simulink model "mdl_SMO_spm_foc_plus_inv"  (R2022b)
settings: Solver=ode3  StartTime=0.0  StopTime=0.4  FixedStep=1e-6  RelTol=1e-3  EnableMultiTasking=on
undefined symbols (not defined in the file): Ls, Rs
libraries: slpidlib x3, spsDCVoltageSourceLib x1, spsGroundLib x1, spsTriangleGeneratorLib x1, spsPermanentMagnetSynchronousMachineLib x1, spsThreePhaseVIMeasurementLib x1, spsUniversalBridgeLib x1, spspowerguiLib x1
settings Model: Creator=jack  LastModifiedBy=jackyeh
settings DebuggingCC: SolverPrmCheckMsg=warning  StateNameClashWarn=warning

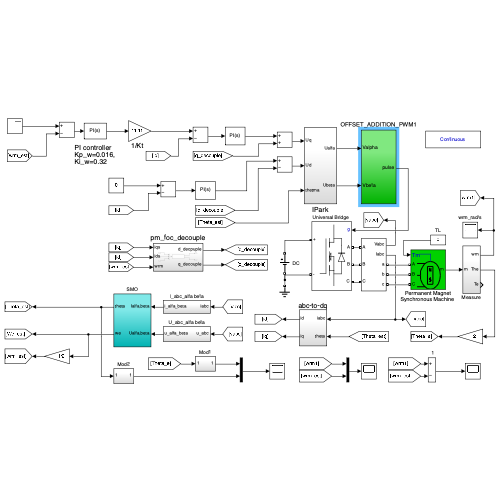
[thumbnail: Simulink's stored preview of the top-level diagram]
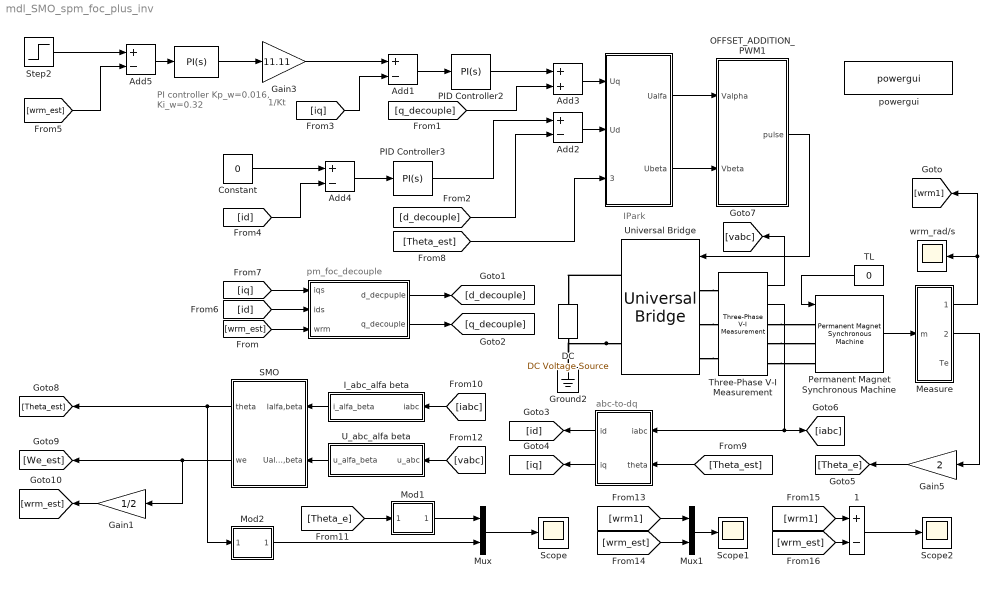
== system mdl_SMO_spm_foc_plus_inv ==
  note: abc-to-dq
  note: IPark
  note: pm_foc_decouple
  note: PI controller
      | Kp_w=0.016, Ki_w=0.32
  note: 1/Kt
  "   " : slpidlib/PID Controller  Controller=PI  Form=Parallel  TimeDomain=Continuous-time  UseExternalTs=off  SampleTime=-1  IntegratorMethod=Forward Euler  FilterMethod=Forward Euler  ControllerParametersSource=internal  P=0.016  I=0.32  UseKiTs=off  D=0  N=100  UseFilter=on  TunerSelectOption=Transfer Function Based (PID Tuner App)  InitialConditionSource=internal  InitialConditionForIntegrator=0  InitialConditionForFilter=0  DifferentiatorICPrevScaledInput=0  ExternalReset=none  TrackingMode=off  Kt=1  LimitOutput=off  SatLimitsSource=internal  UpperSaturationLimit=inf  LowerSaturationLimit=-inf  LinearizeAsGain=on  AntiWindupMode=none  Kb=1  LimitIntegrator=off  UpperIntegratorSaturationLimit=inf  LowerIntegratorSaturationLimit=-inf  POutMin=[]  POutMax=[]  IOutMin=[]  IOutMax=[]  DOutMin=[]  DOutMax=[]  NOutMin=[]  NOutMax=[]  SumOutMin=[]  SumOutMax=[]  SaturationOutMin=[]  SaturationOutMax=[]  PParamMin=[]  PParamMax=[]  IParamMin=[]  IParamMax=[]  DParamMin=[]  DParamMax=[]  NParamMin=[]  NParamMax=[]  KbParamMin=[]  KbParamMax=[]  KtParamMin=[]  KtParamMax=[]  KbOutMin=[]  KbOutMax=[]  KtOutMin=[]  KtOutMax=[]  IntegratorOutMin=[]  IntegratorOutMax=[]  FilterOutMin=[]  FilterOutMax=[]  SumI1OutMin=[]  SumI1OutMax=[]  SumI2OutMin=[]  SumI2OutMax=[]  SumI3OutMin=[]  SumI3OutMax=[]  SumI4OutMin=[]  SumI4OutMax=[]  SumDOutMin=[]  SumDOutMax=[]  DifferentiatorOutMin=[]  DifferentiatorOutMax=[]  FilterDiffOutCoefMin=[]  FilterDiffOutCoefMax=[]  ReciprocalOutMin=[]  ReciprocalOutMax=[]  SumDenOutMin=[]  SumDenOutMax=[]  SumNumOutMin=[]  SumNumOutMax=[]  DivideOutMin=[]  DivideOutMax=[]  UdiffTsProdOutMin=[]  UdiffTsProdOutMax=[]  NTsProdOutMin=[]  NTsProdOutMax=[]  UintegralTsProdOutMin=[]  UintegralTsProdOutMax=[]  UngainTsProdOutMin=[]  UngainTsProdOutMax=[]  ClampingZeroOutDataTypeStr=Inherit: Inherit via back propagation  ClampingZeroOutMin=[]  ClampingZeroOutMax=[]  FilterDenConstantOutDataTypeStr=Inherit: Inherit via back propagation  FilterDenConstantOutMin=[]  FilterDenConstantOutMax=[]  PCopyOutDataTypeStr=Inherit: Inherit via back propagation  PCopyOutMin=[]  PCopyOutMax=[]  NCopyOutDataTypeStr=Inherit: Inherit via back propagation  NCopyOutMin=[]  NCopyOutMax=[]  IntegratorContinuousStateAttributes=''  IntegratorStateMustResolveToSignalObject=off  IntegratorRTWStateStorageClass=Auto  FilterContinuousStateAttributes=''  FilterStateMustResolveToSignalObject=off  FilterRTWStateStorageClass=Auto  ParallelPVariant=InternalParameters  IdealPVariant=Disabled  IVariant=InternalParameters  DVariant=Disabled  IntegratorVariant=Continuous  SatVariant=Disabled  AWVariant=Passthrough  PCopyVariant=Disabled  TRVariant=Disabled  FdbkBlocksVariant=Forward  IdealPFdbkVariant=Disabled  SatFdbkVariant=Disabled  DerivativeFilterVariant=Disabled  NVariant=Disabled  NCopyVariant=Disabled_SignalSpec  FilterICVariant=Disabled  IntegratorICVariant=InternalICs  ExternalResetVariant=Disabled  TRSumVariant=Passthrough  SumFdbkVariant=Disabled  SumVariant=Sum_PI  TsampFilterVariant=InternalTs  TsampNgainVariant=Passthrough  TsampIntegralVariant=Passthrough  ExternalSaturationOutDataTypeStr=Inherit: Same as second input
  "    " : Subsystem
  "     " : Subsystem
  "      " : Subsystem
  "  1" : Sum  Inputs=+-
  Add{1..2,4..5} (4 alike) : Sum  Inputs=+-
  Add3 : Sum
  Constant : Constant  Value=0
  "DC " : spsDCVoltageSourceLib/DC Voltage Source  Amplitude=311  Measurements=None
  Gain1 : Gain  Gain=1/2
  Gain3 : Gain  Gain=11.11
  Gain5 : Gain  Gain=2
  Ground2 : spsGroundLib/Ground  LConnTagsString=a
  I_abc_alfa beta : Subsystem
  Measure : Subsystem
  Mod1 : Subsystem
  Mod2 : Subsystem
  Mux : Mux  Inputs=2
  Mux1 : Mux  Inputs=2
  OFFSET_ADDITION_PWM1 : Subsystem
  PID Controller2 : slpidlib/PID Controller  Controller=PI  Form=Parallel  TimeDomain=Continuous-time  UseExternalTs=off  SampleTime=-1  IntegratorMethod=Forward Euler  FilterMethod=Forward Euler  ControllerParametersSource=internal  P=5.7  I=1200  UseKiTs=off  D=0  N=100  UseFilter=on  TunerSelectOption=Transfer Function Based (PID Tuner App)  InitialConditionSource=internal  InitialConditionForIntegrator=0  InitialConditionForFilter=0  DifferentiatorICPrevScaledInput=0  ExternalReset=none  TrackingMode=off  Kt=1  LimitOutput=off  SatLimitsSource=internal  UpperSaturationLimit=inf  LowerSaturationLimit=-inf  LinearizeAsGain=on  AntiWindupMode=none  Kb=1  LimitIntegrator=off  UpperIntegratorSaturationLimit=inf  LowerIntegratorSaturationLimit=-inf  POutMin=[]  POutMax=[]  IOutMin=[]  IOutMax=[]  DOutMin=[]  DOutMax=[]  NOutMin=[]  NOutMax=[]  SumOutMin=[]  SumOutMax=[]  SaturationOutMin=[]  SaturationOutMax=[]  PParamMin=[]  PParamMax=[]  IParamMin=[]  IParamMax=[]  DParamMin=[]  DParamMax=[]  NParamMin=[]  NParamMax=[]  KbParamMin=[]  KbParamMax=[]  KtParamMin=[]  KtParamMax=[]  KbOutMin=[]  KbOutMax=[]  KtOutMin=[]  KtOutMax=[]  IntegratorOutMin=[]  IntegratorOutMax=[]  FilterOutMin=[]  FilterOutMax=[]  SumI1OutMin=[]  SumI1OutMax=[]  SumI2OutMin=[]  SumI2OutMax=[]  SumI3OutMin=[]  SumI3OutMax=[]  SumI4OutMin=[]  SumI4OutMax=[]  SumDOutMin=[]  SumDOutMax=[]  DifferentiatorOutMin=[]  DifferentiatorOutMax=[]  FilterDiffOutCoefMin=[]  FilterDiffOutCoefMax=[]  ReciprocalOutMin=[]  ReciprocalOutMax=[]  SumDenOutMin=[]  SumDenOutMax=[]  SumNumOutMin=[]  SumNumOutMax=[]  DivideOutMin=[]  DivideOutMax=[]  UdiffTsProdOutMin=[]  UdiffTsProdOutMax=[]  NTsProdOutMin=[]  NTsProdOutMax=[]  UintegralTsProdOutMin=[]  UintegralTsProdOutMax=[]  UngainTsProdOutMin=[]  UngainTsProdOutMax=[]  ClampingZeroOutDataTypeStr=Inherit: Inherit via back propagation  ClampingZeroOutMin=[]  ClampingZeroOutMax=[]  FilterDenConstantOutDataTypeStr=Inherit: Inherit via back propagation  FilterDenConstantOutMin=[]  FilterDenConstantOutMax=[]  PCopyOutDataTypeStr=Inherit: Inherit via back propagation  PCopyOutMin=[]  PCopyOutMax=[]  NCopyOutDataTypeStr=Inherit: Inherit via back propagation  NCopyOutMin=[]  NCopyOutMax=[]  IntegratorContinuousStateAttributes=''  IntegratorStateMustResolveToSignalObject=off  IntegratorRTWStateStorageClass=Auto  FilterContinuousStateAttributes=''  FilterStateMustResolveToSignalObject=off  FilterRTWStateStorageClass=Auto  ParallelPVariant=InternalParameters  IdealPVariant=Disabled  IVariant=InternalParameters  DVariant=Disabled  IntegratorVariant=Continuous  SatVariant=Disabled  AWVariant=Passthrough  PCopyVariant=Disabled  TRVariant=Disabled  FdbkBlocksVariant=Forward  IdealPFdbkVariant=Disabled  SatFdbkVariant=Disabled  DerivativeFilterVariant=Disabled  NVariant=Disabled  NCopyVariant=Disabled_SignalSpec  FilterICVariant=Disabled  IntegratorICVariant=InternalICs  ExternalResetVariant=Disabled  TRSumVariant=Passthrough  SumFdbkVariant=Disabled  SumVariant=Sum_PI  TsampFilterVariant=InternalTs  TsampNgainVariant=Passthrough  TsampIntegralVariant=Passthrough  ExternalSaturationOutDataTypeStr=Inherit: Same as second input
  PID Controller3 : slpidlib/PID Controller  Controller=PI  Form=Parallel  TimeDomain=Continuous-time  UseExternalTs=off  SampleTime=-1  IntegratorMethod=Forward Euler  FilterMethod=Forward Euler  ControllerParametersSource=internal  P=5.7  I=1200  UseKiTs=off  D=0  N=100  UseFilter=on  TunerSelectOption=Transfer Function Based (PID Tuner App)  InitialConditionSource=internal  InitialConditionForIntegrator=0  InitialConditionForFilter=0  DifferentiatorICPrevScaledInput=0  ExternalReset=none  TrackingMode=off  Kt=1  LimitOutput=off  SatLimitsSource=internal  UpperSaturationLimit=inf  LowerSaturationLimit=-inf  LinearizeAsGain=on  AntiWindupMode=none  Kb=1  LimitIntegrator=off  UpperIntegratorSaturationLimit=inf  LowerIntegratorSaturationLimit=-inf  POutMin=[]  POutMax=[]  IOutMin=[]  IOutMax=[]  DOutMin=[]  DOutMax=[]  NOutMin=[]  NOutMax=[]  SumOutMin=[]  SumOutMax=[]  SaturationOutMin=[]  SaturationOutMax=[]  PParamMin=[]  PParamMax=[]  IParamMin=[]  IParamMax=[]  DParamMin=[]  DParamMax=[]  NParamMin=[]  NParamMax=[]  KbParamMin=[]  KbParamMax=[]  KtParamMin=[]  KtParamMax=[]  KbOutMin=[]  KbOutMax=[]  KtOutMin=[]  KtOutMax=[]  IntegratorOutMin=[]  IntegratorOutMax=[]  FilterOutMin=[]  FilterOutMax=[]  SumI1OutMin=[]  SumI1OutMax=[]  SumI2OutMin=[]  SumI2OutMax=[]  SumI3OutMin=[]  SumI3OutMax=[]  SumI4OutMin=[]  SumI4OutMax=[]  SumDOutMin=[]  SumDOutMax=[]  DifferentiatorOutMin=[]  DifferentiatorOutMax=[]  FilterDiffOutCoefMin=[]  FilterDiffOutCoefMax=[]  ReciprocalOutMin=[]  ReciprocalOutMax=[]  SumDenOutMin=[]  SumDenOutMax=[]  SumNumOutMin=[]  SumNumOutMax=[]  DivideOutMin=[]  DivideOutMax=[]  UdiffTsProdOutMin=[]  UdiffTsProdOutMax=[]  NTsProdOutMin=[]  NTsProdOutMax=[]  UintegralTsProdOutMin=[]  UintegralTsProdOutMax=[]  UngainTsProdOutMin=[]  UngainTsProdOutMax=[]  ClampingZeroOutDataTypeStr=Inherit: Inherit via back propagation  ClampingZeroOutMin=[]  ClampingZeroOutMax=[]  FilterDenConstantOutDataTypeStr=Inherit: Inherit via back propagation  FilterDenConstantOutMin=[]  FilterDenConstantOutMax=[]  PCopyOutDataTypeStr=Inherit: Inherit via back propagation  PCopyOutMin=[]  PCopyOutMax=[]  NCopyOutDataTypeStr=Inherit: Inherit via back propagation  NCopyOutMin=[]  NCopyOutMax=[]  IntegratorContinuousStateAttributes=''  IntegratorStateMustResolveToSignalObject=off  IntegratorRTWStateStorageClass=Auto  FilterContinuousStateAttributes=''  FilterStateMustResolveToSignalObject=off  FilterRTWStateStorageClass=Auto  ParallelPVariant=InternalParameters  IdealPVariant=Disabled  IVariant=InternalParameters  DVariant=Disabled  IntegratorVariant=Continuous  SatVariant=Disabled  AWVariant=Passthrough  PCopyVariant=Disabled  TRVariant=Disabled  FdbkBlocksVariant=Forward  IdealPFdbkVariant=Disabled  SatFdbkVariant=Disabled  DerivativeFilterVariant=Disabled  NVariant=Disabled  NCopyVariant=Disabled_SignalSpec  FilterICVariant=Disabled  IntegratorICVariant=InternalICs  ExternalResetVariant=Disabled  TRSumVariant=Passthrough  SumFdbkVariant=Disabled  SumVariant=Sum_PI  TsampFilterVariant=InternalTs  TsampNgainVariant=Passthrough  TsampIntegralVariant=Passthrough  ExternalSaturationOutDataTypeStr=Inherit: Same as second input
  "Permanent Magnet Synchronous Machine " : spsPermanentMagnetSynchronousMachineLib/Permanent Magnet Synchronous Machine  NbPhases=3  FluxDistribution=Sinusoidal  RotorType=Salient-pole  MechanicalLoad=Torque Tm  PresetModel=No  ShowDetailedParameters=on  MeasurementBus=off  Resistance=1.2  Inductance=8.5e-3  dqInductances=[5.7e-3, 5.7e-3]  La=5.7e-3  MachineConstant=Flux linkage established by magnets (V.s)  Flux=0.03  VoltageCst=10.8828  TorqueCst=0.09  Flat=120  Mechanical="[0.00016  0 2]"  PolePairs=4  InitialConditions=[0,0, 0,0]  InitialConditions5ph=[0 0 0 0 0 0]  RefAngle=Aligned with phase A axis (original Park)  IterativeDiscreteModel=Trapezoidal non iterative  TsBlock=-1  TsPowergui=0
  SMO : Subsystem
  Scope : Scope
  Scope1 : Scope
  Scope2 : Scope
  Step2 : Step  Time=0  After=100  SampleTime=0
  TL : Constant  Value=0
  Three-Phase V-I Measurement : spsThreePhaseVIMeasurementLib/Three-Phase V-I Measurement  VoltageMeasurement=phase-to-ground  SetLabelV=off  LabelV=Vabc  Vpu=off  VpuLL=off  CurrentMeasurement=yes  SetLabelI=off  LabelI=Iabc  Ipu=off  Pbase=100e6  Vbase=500e3  OutputType=Complex  PhasorSimulation=off  PSBequivalent=0
  U_abc_alfa beta : Subsystem
  "Universal Bridge " : spsUniversalBridgeLib/Universal Bridge  Arms=3  SnubberResistance=1e5  SnubberCapacitance=inf  Device=MOSFET / Diodes  Ron=1e-3  Lon=0  ForwardVoltages="[  0  0  ]"  ForwardVoltage=0  GTOparameters=[ 10e-6 , 20e-6 ]  IGBTparameters=[ 1e-6 , 2e-6 ]  Measurements=None  Measurements_2=None  converterType=Rectifier
  powergui : spspowerguiLib/powergui  Priority=1  SimulationMode=Continuous  SampleTime=50e-6  frequency=60  Iterations=50  frequencyindice=0  Pbase=100e6  ErrMax=1e-4  UnitsV=kV  UnitsW=MW  buscounter=0  FunctionMessages=off  echomessages=off  EnableUseOfTLC=off  CurrentSourceSwitches=off  DisableSnubberDevices=off  DisableRonSwitches=off  DisableVfSwitches=off  DisplayEquations=off  AutomaticDiscreteSolvers=off  SolverType=Tustin/Backward Euler (TBE)  Interpol=off  ExternalGateDelay=off  methode=off  Ts=100  x0status=blocks  SPID=off  SwTol=0  HookPort=off  NonlinearTolerance=1e-4  nMaxIteration=100  ContinueOnMaxIteration=off  RestoreLinks=warning  ResistiveCurrentMeasurement=off  Frange=[0:2:500]  Ylog=off  Xlog=on  ShowGrid=off  save=off  variable=ZData  structure=0  ZoomFFT=off  StartTime=0.0  cycles=1  DisplayStyle=1  fundamental=60  FreqAxis=off  MaxFrequency=1000  frequencyindicesteady=1  RmsSteady=1  display=off
  wrm_rad/s : Scope
  wires:
  "   "/1 -> Gain3/1
  Add1/1 -> PID Controller2/1
  Constant/1 -> Add4/1
  Add4/1 -> PID Controller3/1
  Add5/1 -> "   "/1
  "Permanent Magnet Synchronous Machine "/1 -> Measure/1(m)
  OFFSET_ADDITION_PWM1/1(pulse) -> "Universal Bridge "/1
  "     "/1(Ualfa) -> OFFSET_ADDITION_PWM1/1(Valpha)
  "     "/2(Ubeta) -> OFFSET_ADDITION_PWM1/2(Vbeta)
  Three-Phase V-I Measurement/2 -> [iabc], "      "/1(iabc)
  Measure/2(The) -> Gain5/1
  Measure/1(wm) -> [wrm1], wrm_rad/s/1
  PID Controller3/1 -> Add2/1
  PID Controller2/1 -> Add3/1
  Add3/1 -> "     "/1(Uq)
  Add2/1 -> "     "/2(Ud)
  [wrm_est] -> "    "/3(wrm)
  Gain3/1 -> Add1/1
  Step2/1 -> Add5/1
  TL/1 -> "Permanent Magnet Synchronous Machine "/1
  "    "/1(d_decpuple) -> [d_decouple]
  "    "/2(q_decouple) -> [q_decouple]
  "      "/1(id) -> [id]
  "      "/2(iq) -> [iq]
  [iq] -> Add1/2
  [id] -> Add4/2
  [wrm_est] -> Add5/2
  [iq] -> "    "/1(iqs)
  [id] -> "    "/2(ids)
  [Theta_est] -> "     "/3(thetma)
  [Theta_est] -> "      "/2(theta)
  I_abc_alfa beta/1(i_alfa_beta) -> SMO/1(Ialfa,beta)
  U_abc_alfa beta/1(u_alfa_beta) -> SMO/2(Ualfa,beta)
  Three-Phase V-I Measurement/1 -> [vabc]
  [iabc] -> I_abc_alfa beta/1(iabc)
  [vabc] -> U_abc_alfa beta/1(u_abc)
  SMO/2(we) -> Gain1/1, [We_est]
  Gain1/1 -> [wrm_est]
  Mux/1 -> Scope/1
  Gain5/1 -> [Theta_e]
  [q_decouple] -> Add3/2
  [d_decouple] -> Add2/2
  SMO/1(theta) -> [Theta_est], Mod2/1(In1)
  [Theta_e] -> Mod1/1(In1)
  Mod1/1(Out1) -> Mux/1
  [wrm1] -> Mux1/1
  [wrm_est] -> Mux1/2
  Mux1/1 -> Scope1/1
  [wrm1] -> "  1"/1
  [wrm_est] -> "  1"/2
  "  1"/1 -> Scope2/1
  Mod2/1(Out1) -> Mux/2
  connections:
  "Universal Bridge "/RConn2 -- Ground2/LConn1 -- "DC "/LConn1
  "Universal Bridge "/LConn1 -- Three-Phase V-I Measurement/LConn1
  "Universal Bridge "/LConn3 -- Three-Phase V-I Measurement/LConn3
  Three-Phase V-I Measurement/RConn3 -- "Permanent Magnet Synchronous Machine "/LConn3
  Three-Phase V-I Measurement/RConn1 -- "Permanent Magnet Synchronous Machine "/LConn1
  Three-Phase V-I Measurement/RConn2 -- "Permanent Magnet Synchronous Machine "/LConn2
  "Universal Bridge "/RConn1 -- "DC "/RConn1
  "Universal Bridge "/LConn2 -- Three-Phase V-I Measurement/LConn2

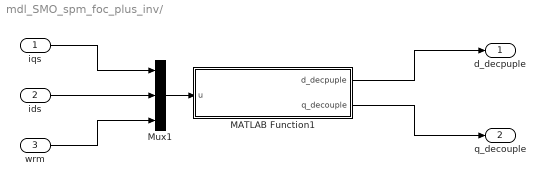
== system mdl_SMO_spm_foc_plus_inv/     ==
  iqs : Inport
  ids : Inport  Port=2
  wrm : Inport  Port=3
  MATLAB Function1 : MATLAB Function  TreatAsAtomicUnit=on
  Mux1 : Mux  Inputs=3
  d_decpuple : Outport
  q_decouple : Outport  Port=2
  wires:
  iqs/1 -> Mux1/1
  MATLAB Function1/1(d_decpuple) -> d_decpuple/1
  ids/1 -> Mux1/2
  Mux1/1 -> MATLAB Function1/1(u)
  MATLAB Function1/2(q_decouple) -> q_decouple/1
  wrm/1 -> Mux1/3

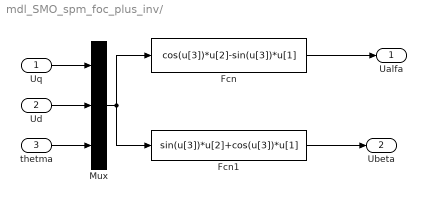
== system mdl_SMO_spm_foc_plus_inv/      ==
  Uq : Inport
  Ud : Inport  Port=2
  thetma : Inport  Port=3
  Fcn : Fcn  Expr=cos(u[3])*u[2]-sin(u[3])*u[1]
  Fcn1 : Fcn  Expr=sin(u[3])*u[2]+cos(u[3])*u[1]
  Mux : Mux  Inputs=3
  Ualfa : Outport
  Ubeta : Outport  Port=2
  wires:
  Uq/1 -> Mux/1
  Ud/1 -> Mux/2
  thetma/1 -> Mux/3
  Mux/1 -> Fcn/1, Fcn1/1
  Fcn/1 -> Ualfa/1
  Fcn1/1 -> Ubeta/1

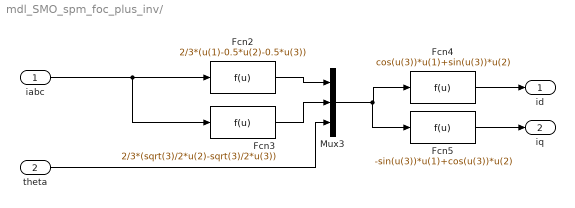
== system mdl_SMO_spm_foc_plus_inv/       ==
  iabc : Inport
  theta : Inport  Port=2
  Fcn2 : Fcn  Expr=2/3*(u(1)-0.5*u(2)-0.5*u(3))
  Fcn3 : Fcn  Expr=2/3*(sqrt(3)/2*u(2)-sqrt(3)/2*u(3))
  Fcn4 : Fcn  Expr=cos(u(3))*u(1)+sin(u(3))*u(2)
  Fcn5 : Fcn  Expr=-sin(u(3))*u(1)+cos(u(3))*u(2)
  Mux3 : Mux  Inputs=3
  id : Outport
  iq : Outport  Port=2
  wires:
  iabc/1 -> Fcn3/1, Fcn2/1
  Fcn2/1 -> Mux3/1
  Fcn3/1 -> Mux3/2
  theta/1 -> Mux3/3
  Mux3/1 -> Fcn5/1, Fcn4/1
  Fcn4/1 -> id/1
  Fcn5/1 -> iq/1

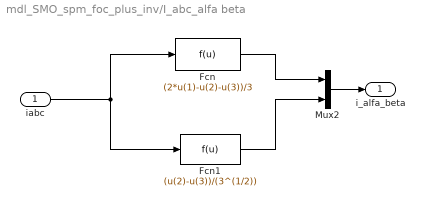
== system mdl_SMO_spm_foc_plus_inv/I_abc_alfa beta ==
  iabc : Inport
  Fcn : Fcn  Expr=(2*u(1)-u(2)-u(3))/3
  Fcn1 : Fcn  Expr=(u(2)-u(3))/(3^(1/2))
  Mux2 : Mux  Inputs=2
  i_alfa_beta : Outport
  wires:
  iabc/1 -> Fcn/1, Fcn1/1
  Mux2/1 -> i_alfa_beta/1
  Fcn/1 -> Mux2/1
  Fcn1/1 -> Mux2/2

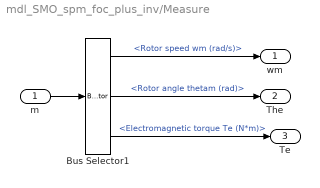
== system mdl_SMO_spm_foc_plus_inv/Measure ==
  m : Inport
  Bus Selector1 : BusSelector  OutputSignals=Rotor speed wm (rad/s),Rotor angle thetam (rad),Electromagnetic torque Te (N*m)
  wm : Outport
  The : Outport  Port=2
  Te : Outport  Port=3
  wires:
  Bus Selector1/2 -> The/1  "<Rotor angle thetam (rad)>"
  Bus Selector1/3 -> Te/1  "<Electromagnetic torque Te (N*m)>"
  m/1 -> Bus Selector1/1
  Bus Selector1/1 -> wm/1  "<Rotor speed wm (rad/s)>"

== system mdl_SMO_spm_foc_plus_inv/Mod1 ==
  In1 : Inport
  Constant1 : Constant  Value=pi
  Math Function : Math  Operator=mod  SignedPower=on
  Out1 : Outport
  wires:
  In1/1 -> Math Function/1
  Math Function/1 -> Out1/1
  Constant1/1 -> Math Function/2

== system mdl_SMO_spm_foc_plus_inv/Mod2 ==
  In1 : Inport
  Constant1 : Constant  Value=pi
  Math Function : Math  Operator=mod  SignedPower=on
  Out1 : Outport
  wires:
  Constant1/1 -> Math Function/2
  Math Function/1 -> Out1/1
  In1/1 -> Math Function/1

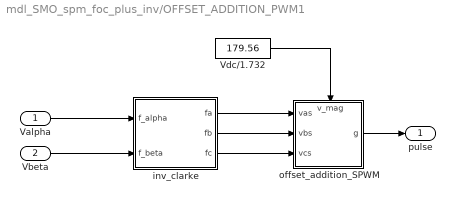
== system mdl_SMO_spm_foc_plus_inv/OFFSET_ADDITION_PWM1 ==
  Valpha : Inport
  Vbeta : Inport  Port=2
  Vdc/1.732 : Constant  Value=179.56
  inv_clarke : Subsystem
  offset_addition_SPWM : Subsystem
      settings: PortSchema="{\"entries\":[{\"content\":{\"sides\":[{\"content\":{\"connectorIds\":[\"In1\",\"In2\",\"In3\"]},\"type\":\"ConnectorPlacement.EquallySpacedRectSide\",\"uuid\":\"bd7bea3a-7add-49ec-8b52-f68dbb33beea\"},{\"content\":{\"connectorIds\":[\"Out1\"],\"side\":\"RIGHT\"},\"type\":\"ConnectorPlacement.EquallySpacedRectSide\",\"uuid\":\"aa5e81bc-27af-49d7-8d73-7e78ac021e04\"},{\"content\":{\"connectorIds\":[\"In4\"],\"side\":\"TOP\"},\"type\":\"ConnectorPlacement.EquallySpacedRectSide\",\"uuid\":\"5bcd18e6-6f27-4bab-991b-2041f8ef0a25\"}]},\"type\":\"ConnectorPlacement.EquallySpacedConnector\",\"uuid\":\"27ed4ada-ba8b-4440-bbdb-1c3a657b0505\"}],\"packageUris\":[\"http://schema.mathworks.com/mf0/Connector/R2020b\"],\"version\":\"1.0\"}"
  pulse : Outport
  wires:
  Valpha/1 -> inv_clarke/1(f_alpha)
  Vbeta/1 -> inv_clarke/2(f_beta)
  inv_clarke/1(fa) -> offset_addition_SPWM/1(vas)
  inv_clarke/2(fb) -> offset_addition_SPWM/2(vbs)
  inv_clarke/3(fc) -> offset_addition_SPWM/3(vcs)
  offset_addition_SPWM/1(g) -> pulse/1
  Vdc/1.732/1 -> offset_addition_SPWM/4(v_mag)

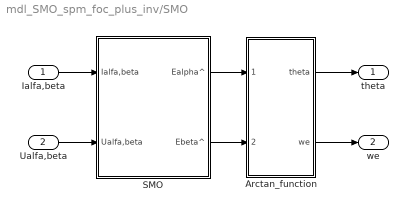
== system mdl_SMO_spm_foc_plus_inv/SMO ==
  Ialfa,beta : Inport
  Ualfa,beta : Inport  Port=2
  Arctan_function : Subsystem
  SMO : Subsystem
  theta : Outport
  we : Outport  Port=2
  wires:
  Ualfa,beta/1 -> SMO/2(Ualfa,beta)
  Ialfa,beta/1 -> SMO/1(Ialfa,beta)
  SMO/1(Ealpha^) -> Arctan_function/1(Ealpha^)
  SMO/2(Ebeta^) -> Arctan_function/2(Ebeta^)
  Arctan_function/1(theta) -> theta/1
  Arctan_function/2(we) -> we/1

== system mdl_SMO_spm_foc_plus_inv/U_abc_alfa beta ==
  u_abc : Inport
  Fcn : Fcn  Expr=(2*u(1)-u(2)-u(3))/3
  Fcn1 : Fcn  Expr=(u(2)-u(3))/(3^(1/2))
  Mux2 : Mux  Inputs=2
  u_alfa_beta : Outport
  wires:
  u_abc/1 -> Fcn/1, Fcn1/1
  Mux2/1 -> u_alfa_beta/1
  Fcn/1 -> Mux2/1
  Fcn1/1 -> Mux2/2

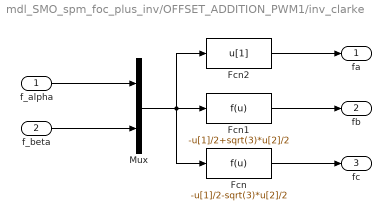
== system mdl_SMO_spm_foc_plus_inv/OFFSET_ADDITION_PWM1/inv_clarke ==
  f_alpha : Inport
  f_beta : Inport  Port=2
  Fcn : Fcn  Expr=-u[1]/2-sqrt(3)*u[2]/2
  Fcn1 : Fcn  Expr=-u[1]/2+sqrt(3)*u[2]/2
  Fcn2 : Fcn  Expr=u[1]
  Mux : Mux  Inputs=2
  fa : Outport
  fb : Outport  Port=2
  fc : Outport  Port=3
  wires:
  Mux/1 -> Fcn2/1, Fcn1/1, Fcn/1
  f_alpha/1 -> Mux/1
  f_beta/1 -> Mux/2
  Fcn2/1 -> fa/1
  Fcn1/1 -> fb/1
  Fcn/1 -> fc/1

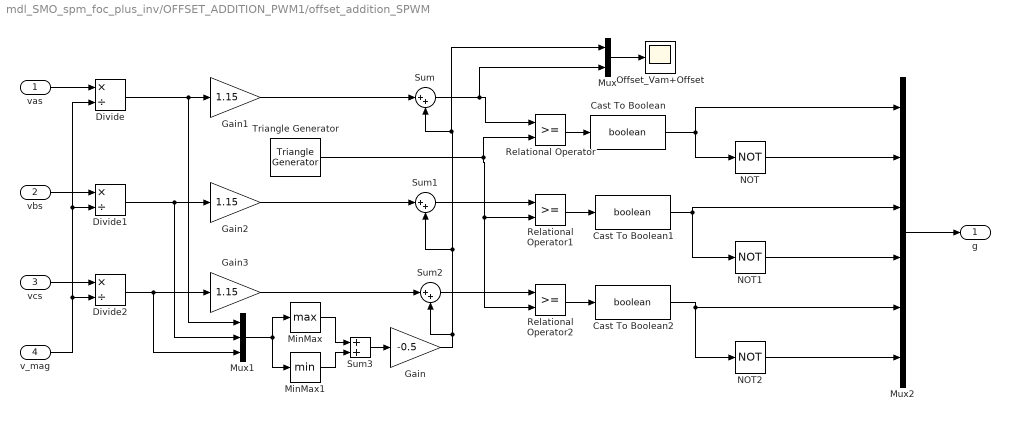
== system mdl_SMO_spm_foc_plus_inv/OFFSET_ADDITION_PWM1/offset_addition_SPWM ==
  vas : Inport
  vbs : Inport  Port=2
  vcs : Inport  Port=3
  v_mag : Inport  Port=4
  Cast To Boolean : DataTypeConversion  OutDataTypeStr=boolean  SaturateOnIntegerOverflow=off  RndMeth=Floor
  Cast To Boolean1 : DataTypeConversion  OutDataTypeStr=boolean  SaturateOnIntegerOverflow=off  RndMeth=Floor
  Cast To Boolean2 : DataTypeConversion  OutDataTypeStr=boolean  SaturateOnIntegerOverflow=off  RndMeth=Floor
  Divide : Product  Inputs=*/
  Divide1 : Product  Inputs=*/
  Divide2 : Product  Inputs=*/
  Gain : Gain  Gain=-0.5
  Gain1 : Gain  Gain=1.15
  Gain2 : Gain  Gain=1.15
  Gain3 : Gain  Gain=1.15
  MinMax : MinMax  Function=max
  MinMax1 : MinMax
  Mux : Mux  Inputs=2
  Mux1 : Mux  Inputs=3
  Mux2 : Mux  Inputs=6
  NOT : Logic  Operator=NOT  IconShape=distinctive  AllPortsSameDT=off  OutDataTypeStr=boolean
  NOT1 : Logic  Operator=NOT  IconShape=distinctive  AllPortsSameDT=off  OutDataTypeStr=boolean
  NOT2 : Logic  Operator=NOT  IconShape=distinctive  AllPortsSameDT=off  OutDataTypeStr=boolean
  Offset_Vam+Offset : Scope
  Relational Operator : RelationalOperator  OutDataTypeStr=boolean  RndMeth=Simplest  InputSameDT=off
  Relational Operator1 : RelationalOperator  OutDataTypeStr=boolean  RndMeth=Simplest  InputSameDT=off
  Relational Operator2 : RelationalOperator  OutDataTypeStr=boolean  RndMeth=Simplest  InputSameDT=off
  Sum : Sum  Inputs=|++
  Sum1 : Sum  Inputs=|++
  Sum2 : Sum  Inputs=|++
  Sum3 : Sum
  Triangle Generator : spsTriangleGeneratorLib/Triangle Generator  Freq=10000  Phase=90  Ts=0
  g : Outport
  wires:
  NOT/1 -> Mux2/2
  Relational Operator/1 -> Cast To Boolean/1
  Cast To Boolean/1 -> Mux2/1, NOT/1
  Triangle Generator/1 -> Relational Operator2/2, Relational Operator1/2, Relational Operator/2
  Relational Operator1/1 -> Cast To Boolean1/1
  Cast To Boolean1/1 -> Mux2/3, NOT1/1
  Relational Operator2/1 -> Cast To Boolean2/1
  NOT2/1 -> Mux2/6
  Cast To Boolean2/1 -> Mux2/5, NOT2/1
  Sum/1 -> Mux/2, Relational Operator/1
  Sum1/1 -> Relational Operator1/1
  Sum2/1 -> Relational Operator2/1
  Gain/1 -> Sum2/2, Sum1/2, Mux/1, Sum/2
  Mux1/1 -> MinMax1/1, MinMax/1
  MinMax/1 -> Sum3/1
  MinMax1/1 -> Sum3/2
  Sum3/1 -> Gain/1
  Mux/1 -> Offset_Vam+Offset/1
  vas/1 -> Divide/1
  v_mag/1 -> Divide/2, Divide1/2, Divide2/2
  vbs/1 -> Divide1/1
  vcs/1 -> Divide2/1
  Divide/1 -> Mux1/1, Gain1/1
  Divide1/1 -> Mux1/2, Gain2/1
  Divide2/1 -> Mux1/3, Gain3/1
  NOT1/1 -> Mux2/4
  Mux2/1 -> g/1
  Gain1/1 -> Sum/1
  Gain2/1 -> Sum1/1
  Gain3/1 -> Sum2/1

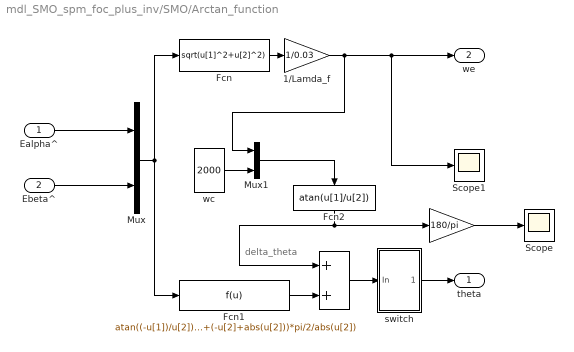
== system mdl_SMO_spm_foc_plus_inv/SMO/Arctan_function ==
  note: delta_theta
  Ealpha^ : Inport
  Ebeta^ : Inport  Port=2
  "  " : Sum
  "    " : Gain  Gain=180/pi
  1/Lamda_f : Gain  Gain=1/0.03
  Fcn : Fcn  Expr=sqrt(u[1]^2+u[2]^2)
  Fcn1 : Fcn  Expr=atan((-u[1])/u[2])+(-u[2]+abs(u[2]))*pi/2/abs(u[2])
  Fcn2 : Fcn  Expr=atan(u[1]/u[2])
  Mux : Mux  Inputs=2
  Mux1 : Mux  Inputs=2
  Scope : Scope
  Scope1 : Scope
  switch : Subsystem
  wc : Constant  Value=2000
  theta : Outport
  we : Outport  Port=2
  wires:
  Mux/1 -> Fcn/1, Fcn1/1
  Fcn/1 -> 1/Lamda_f/1
  1/Lamda_f/1 -> Mux1/1, Scope1/1, we/1
  Fcn1/1 -> "  "/2
  "  "/1 -> switch/1(In)
  Ebeta^/1 -> Mux/2
  Ealpha^/1 -> Mux/1
  switch/1(theta) -> theta/1
  Fcn2/1 -> "  "/1, "    "/1
  wc/1 -> Mux1/2
  Mux1/1 -> Fcn2/1
  "    "/1 -> Scope/1

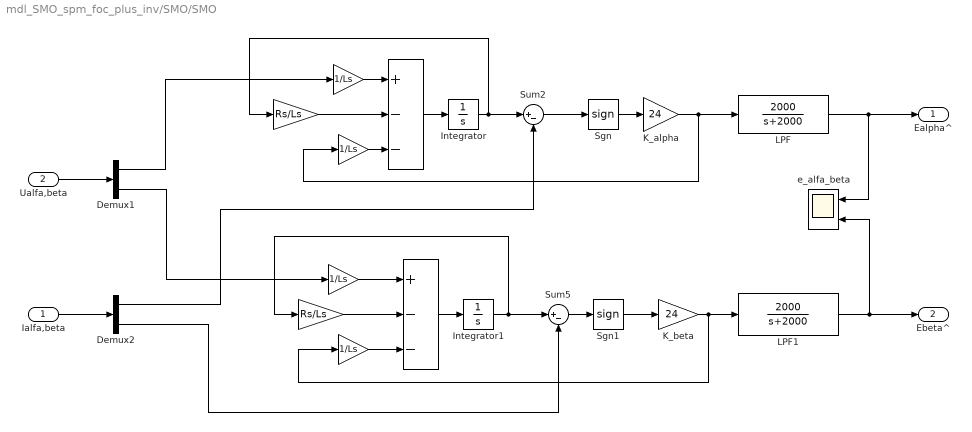
== system mdl_SMO_spm_foc_plus_inv/SMO/SMO ==
  Ialfa,beta : Inport
  Ualfa,beta : Inport  Port=2
  " " : Sum  Inputs=+--
  "  " : Gain  Gain=1/Ls
  "   " : Sum  Inputs=+--
  "    " : Gain  Gain=Rs/Ls
  "     " : Gain  Gain=1/Ls
  "       " : Gain  Gain=1/Ls
  "        " : Gain  Gain=Rs/Ls
  "          " : Gain  Gain=1/Ls
  Demux1 : Demux  Outputs=2
  Demux2 : Demux  Outputs=2
  Integrator : Integrator
  Integrator1 : Integrator
  K_alpha : Gain  Gain=24
  "K_beta " : Gain  Gain=24
  LPF : TransferFcn  Numerator=[2000]  Denominator=[1 2000]
  LPF1 : TransferFcn  Numerator=[2000]  Denominator=[1 2000]
  Sgn : Signum  ZeroCross=off
  Sgn1 : Signum  ZeroCross=off
  Sum2 : Sum  Inputs=|+-
  Sum5 : Sum  Inputs=|+-
  e_alfa_beta : Scope  NumInputPorts=2
  Ealpha^ : Outport
  Ebeta^ : Outport  Port=2
  wires:
  Integrator/1 -> Sum2/1, "    "/1
  Sgn/1 -> K_alpha/1
  K_alpha/1 -> "  "/1, LPF/1
  Integrator1/1 -> Sum5/1, "        "/1
  Sum5/1 -> Sgn1/1
  Sgn1/1 -> "K_beta "/1
  "K_beta "/1 -> "          "/1, LPF1/1
  Demux2/1 -> Sum2/2
  Demux2/2 -> Sum5/2
  "     "/1 -> " "/1
  "    "/1 -> " "/2
  "  "/1 -> " "/3
  " "/1 -> Integrator/1
  Demux1/2 -> "       "/1
  "       "/1 -> "   "/1
  "        "/1 -> "   "/2
  "   "/1 -> Integrator1/1
  "          "/1 -> "   "/3
  Sum2/1 -> Sgn/1
  LPF1/1 -> e_alfa_beta/2, Ebeta^/1
  LPF/1 -> Ealpha^/1, e_alfa_beta/1
  Demux1/1 -> "     "/1
  Ialfa,beta/1 -> Demux2/1
  Ualfa,beta/1 -> Demux1/1

== system mdl_SMO_spm_foc_plus_inv/SMO/Arctan_function/switch ==
  In : Inport
  Constant4 : Constant  Value=0
  Step1 : Step  Time=0.001  SampleTime=0
  Switch : Switch  Threshold=1  SaturateOnIntegerOverflow=off  InputSameDT=off
  theta : Outport
  wires:
  Step1/1 -> Switch/2
  Constant4/1 -> Switch/3
  In/1 -> Switch/1
  Switch/1 -> theta/1

== matlab function mdl_SMO_spm_foc_plus_inv/    /MATLAB Function1 ==
  data: u input; d_decpuple output; q_decouple output
function [d_decpuple, q_decouple] = decouple(u)
    Ld = 0.0057;
    Lq = 0.0057;
    Lamda_f = 0.03;
    pole = 4;
    wr = u(3)*pole/2;
    d_decpuple = Ld*(wr*(Lq/Ld)*u(1));
    q_decouple = Lq*(wr*(Ld*u(2)+Lamda_f)/Lq);
